simulink model "BEV_Laengsdynamikmodell_Reiter"  (R2022b)
settings: Solver=FixedStepAuto  StartTime=0.0  StopTime=1068  FixedStep=0.001  MaxStep=0.1  RelTol=1e-3  EnableMultiTasking=on
model workspace (MAT data in the model file):
  BTMSConfig.BTMS_included = 1
  BTMSConfig.T_fluid = 20
  BTMSConfig.Vdot_BTMS = 0.0045
  BTMSConfig.channel_def_mat = [1  2  3  0  0  0; 334  335  336  0  0  0; 10  11  12  13  14  15; 19  20  21  22  23  24; 28  29  30  31  32  33; 52  53  54  55  56  57; 61  62  63  64  65  66; 70  71  72  73  74  75; 94  95  96  97  98  99; 103  104  105  106  107  108; 112  113  114  115  116  117; 136  137  138  139  140  141; 145  146  147  148  149  150; 154  155  156  157  158  159; 178  179  180  181  182  183; 187  188  189  190  191  192; 196  197  198  199  200  201; 220  221  222  223  224  225; 229  230  231  232  233  234; 238  239  240  241  242  243; 262  263  264  265  266  267; 271  272  273  274  275  276; 280  281  282  283  284  285; 304  305  306  307  308  309; 313  314  315  316  317  318; 322  323  324  325  326  327]
  BTMSConfig.channel_num_adj_cells = [3 3 6 6 6 6 6 6 6 6 6 6 6 6 6 6 6 6 6 6 6 6 6 6 6 6]
  BTMSConfig.num_channels = 26
  BTMSConfig.channel_length = [1.03690125; 1.03690125; 1.03690125; 1.03690125; 1.03690125; 1.03690125; 1.03690125; 1.03690125; 1.03690125; 1.03690125; 1.03690125; 1.03690125; 1.03690125; 1.03690125; 1.03690125; 1.03690125; 1.03690125; 1.03690125; 1.03690125; 1.03690125; 1.03690125; 1.03690125; 1.03690125; 1.03690125; 1.03690125; 1.03690125]
  BTMSConfig.channel_mdot = [0.184314576259; 0.184314576259; 0.184314576259; 0.184314576259; 0.184314576259; 0.184314576259; 0.184314576259; 0.184314576259; 0.184314576259; 0.184314576259; 0.184314576259; 0.184314576259; 0.184314576259; 0.184314576259; 0.184314576259; 0.184314576259; 0.184314576259; 0.184314576259; 0.184314576259; 0.184314576259; 0.184314576259; 0.184314576259; 0.184314576259; 0.184314576259; 0.184314576259; 0.184314576259]
  BTMSConfig.fluid_para.kin_vis = 3.46803646108e-06
  BTMSConfig.fluid_para.lambda = 0.389148353131
  BTMSConfig.fluid_para.rho = 1064.92866283
  BTMSConfig.fluid_para.cp = 3312.04190374
  BTMSConfig.fluid_para.Pr = 31.4329250552
  BTMSConfig.lambda_wall = 236
  BTMSConfig.channel_alpha = [597.661290321; 597.661290321; 668.795841133; 668.795841133; 668.795841133; 668.795841133; 668.795841133; 668.795841133; 668.795841133; 668.795841133; 668.795841133; 668.795841133; 668.795841133; 668.795841133; 668.795841133; 668.795841133; 668.795841133; 668.795841133; 668.795841133; 668.795841133; 668.795841133; 668.795841133; 668.795841133; 668.795841133; 668.795841133; 668.795841133]
  BTMSConfig.channel_orientation = [120 120 120 120 120 120 120 120 120 120 120 120 120 120 120 120 120 120 120 120 120 120 120 120 120 120]
  BatPara.electrical.C_A = 73.6
  BatPara.electrical.OCV.U = [3.071 3.168 3.237 3.287 3.317 3.326 3.333 3.339 3.346 3.352 3.36 3.407 3.46 3.504 3.537 3.56 3.581 3.601 3.621 3.645 3.672 3.707 3.767 3.806 3.84 3.872 3.904 3.938 3.978 4.024 4.068 4.086 4.103 4.122 4.148 4.184]
  BatPara.electrical.OCV.SOC = [-1.355e-05 0.0099 0.0199 0.0299 0.0399 0.0499 0.0599 0.0699 0.0799 0.0899 0.0999 0.1399 0.1799 0.2199 0.2599 0.2999 0.3399 0.3799 0.4199 0.4599 0.4999 0.5399 0.5799 0.6199 0.6599 0.6999 0.7399 0.7799 0.8199 0.8599 0.8999 0.9199 0.9399 0.9599 0.9799 0.9999]
  BatPara.electrical.OCV.U_hyst = [0 0.0139 0.0165 0.0207 0.0196 0.0154 0.01449 0.0144 0.0144 0.0156 0.0186 0.0265 0.027 0.0307 0.0202 0.0156 0.0144 0.0144 0.0148 0.0162 0.0173 0.0171 0.0167 0.0148 0.0135 0.012 0.0112 0.0116 0.0122 0.0116 0.0095 0.008 0.0066 0.0062 0.004 -0.0013]
  BatPara.electrical.OCV.beta_hyst = 0.004
  BatPara.electrical.dyn.SOC = [0 0.1 0.2 0.3 0.4 0.5 0.6 0.7 0.8 0.9 1]
  BatPara.electrical.dyn.T = [8 25]
  BatPara.electrical.dyn.C_rate = [-1 1]
  BatPara.electrical.dyn.R_0 = reshape([0.00126739565217 0.00123344755435 0.00124099157609 0.00122590353261 0.00119195543478 0.00121081548913 0.0012145875 0.00118063940217 0.00116932336957 0.00118441141304 0.00121835951087 0.001041075 0.00101844293478 0.00101467092391 0.000995810869565 0.00100712690217 0.00100712690217 0.0010033548913 0.000995810869565 0.000999582880435 0.000999582880435 0.00101467092391 0.00126739565217 0.00123344755435 0.00123721956522 0.00124853559783 0.0012145875 0.00121835951087 0.00120327146739 0.00115423532609 0.00111651521739 0.00116177934783 0.00124853559783 0.00101844293478 0.0010033548913 0.000988266847826 0.000980722826087 0.000999582880435 0.00100712690217 0.000992038858696 0.000988266847826 0.000992038858696 0.000992038858696 0.00103353097826], [11 2 2])
  BatPara.electrical.dyn.RC1_enable = 1
  BatPara.electrical.dyn.R1 = reshape([0.00305155679348 0.00184074130435 0.000543169565217 0.0005205375 0.000535625543478 0.00052430951087 0.000595977717391 0.000675189945652 0.000656329891304 0.000671417934783 0.00310813695652 0.00144845217391 0.00026404076087 0.000324392934783 0.000441325271739 0.00043755326087 0.000467729347826 0.000543169565217 0.000577117663043 0.000622381793478 0.000716682065217 0.000392289130435 0.00228583858696 0.000531853532609 0.000558257608696 0.0005205375 0.000535625543478 0.000528081521739 0.000599749728261 0.000588433695652 0.000573345652174 0.00078457826087 0.00527327119565 0.00043000923913 0.000497905434783 0.000562029619565 0.000471501358696 0.00043000923913 0.000467729347826 0.000531853532609 0.000550713586957 0.000645013858696 0.000347025 0.00200293777174], [11 2 2])
  BatPara.electrical.dyn.C1 = reshape([479.653973057 217.512628773 46.5003962251 42.831265759 41.5216194799 46.4844895901 51.8132123046 53.3853180607 49.1037821483 56.1530725452 111.221842807 262.053857791 81.8714501837 106.455154528 100.415935451 100.681046034 103.313594121 101.874043657 100.628023918 97.120610907 102.99015921 115.718118291 136.505439089 54.5809667891 52.1048339457 51.0443916144 48.1758951084 49.1170376774 50.7023989626 41.7018946762 34.2814494633 86.0389885455 157.18936676 95.0819105252 125.646509617 106.444550104 88.175779843 87.666767524 98.570765795 90.2781067646 87.6057920899 95.423903177 88.220848642 173.719011599], [11 2 2])
  BatPara.electrical.dyn.RC2_enable = 1
  BatPara.electrical.dyn.R2 = reshape([0.0371128149457 0.00761568994565 0.00188223342391 0.00149371630435 0.00124099157609 0.00113914728261 0.00121835951087 0.00130888777174 0.0014371361413 0.00179170516304 0.00087133451087 0.00198784972826 0.00157292853261 0.000788350271739 0.000279128804348 0.000147108423913 0.000101844293478 0.000147108423913 0.000154652445652 0.000211232608696 0.000463957336957 0.00153143641304 0.00158801657609 0.00150503233696 0.00138432798913 0.0011768673913 0.00102598695652 0.000992038858696 0.0010901111413 0.00123344755435 0.0014371361413 0.0023801388587 0.00301760869565 0.00110142717391 0.000769490217391 0.000324392934783 0.000203688586957 0.000132020380435 8.29842391304e-05 0.000139564402174 0.000143336413043 0.0001735125 0.000943002717391 0.00147108423913], [11 2 2])
  BatPara.electrical.dyn.C2 = reshape([1973.40894748 900.304934803 341.260946618 299.415892227 291.865542828 295.05482314 288.522498379 273.085109142 245.8184857 221.216223615 7420.2702399 6327.38897774 467.140753548 432.665773359 969.97334486 2103.52257042 4757.71958793 4941.24503998 4682.62966645 2433.97495858 823.399005835 207.488797637 8423.5149629 263.172624451 257.859808371 259.540609466 269.651927095 270.137079461 266.825848282 219.021107989 196.134111375 206.189755781 753.934730927 364.492586989 467.445630718 1063.18622578 1300.61131042 2191.47565737 6693.27604639 4673.61590663 3457.28059938 2977.36946906 249.909141993 598.921922052], [11 2 2])
  BatPara.electrical.dyn.RC3_enable = 1
  BatPara.electrical.dyn.R3 = reshape([0.0586321369565 0.00301760869565 0.00136169592391 0.000377201086957 0.000245180706522 0.000237636684783 0.000354569021739 0.000418693206522 0.000414921195652 0.000543169565217 0.00268944375 0.0130285255435 0.00200293777174 0.000305532880435 0.000207460597826 0.000199916576087 0.000218776630435 0.000294216847826 0.000282900815217 0.000294216847826 0.000396061141304 0.000716682065217 0.00111274320652 0.000988266847826 0.000467729347826 0.000309304891304 0.000267812771739 0.00025649673913 0.000445097282609 0.000354569021739 0.000331936956522 0.000667645923913 0.00183319728261 0.000973178804348 0.000550713586957 0.000297988858696 0.000226320652174 0.000203688586957 0.000218776630435 0.000316848913043 0.000286672826087 0.000294216847826 0.000320620923913 0.000912826630435], [11 2 2])
  BatPara.electrical.dyn.C3 = reshape([1248.67084504 11155.8533247 2688.2213097 10360.5215763 20766.1119516 25866.8395649 25835.0262949 18441.0921403 17529.1117355 14689.7773936 21614.4658166 967.65362726 1686.10330668 11397.103955 28173.3016353 32765.0169296 33814.8548375 30797.8964052 26280.4120741 23409.2644622 20198.7753044 17645.7603919 110580.275196 12033.3693538 21842.4609178 32287.8178806 35262.3586197 33658.4395937 24832.9082919 30169.5843239 23600.1440818 8825.53130178 4782.59491391 11481.9393415 18952.7555652 32881.6655861 35774.0220445 36179.6412362 36784.093365 33279.3314603 34679.1153375 30267.6752395 14806.42605 10532.8434551], [11 2 2])
  BatPara.electrical.dyn.RC4_enable = 1
  BatPara.electrical.dyn.R4 = reshape([0.00299120461957 0.00170494891304 0.00207460597826 0.00211609809783 0.00188600543478 0.00175398505435 0.00305910081522 0.00309682092391 0.00262909157609 0.00293085244565 0.0235524358696 0.00224811847826 0.0018596013587 0.0014258201087 0.00130888777174 0.00113914728261 0.00103730298913 0.00235750679348 0.00175775706522 0.00150880434783 0.00162573668478 0.0036060423913 0.00636715434783 0.00329296548913 0.00247066711957 0.00219531032609 0.00185205733696 0.00163328070652 0.00284786820652 0.00268944375 0.00252724728261 0.00311190896739 0.00737805326087 0.00293839646739 0.00196144565217 0.00135792391304 0.00102975896739 0.0008675625 0.000886422554348 0.0019576736413 0.00150503233696 0.0014258201087 0.00169363288043 0.00431895244565], [11 2 2])
  BatPara.electrical.dyn.C4 = reshape([24482.9623226 39292.0394784 29930.9847994 32009.4517686 34382.1914848 35206.6853973 29949.5425402 24546.5888625 25394.9427275 24239.0605864 85967.4086881 14848.8437432 27059.8371875 39573.0566962 47080.9884014 52152.5538506 55116.4901664 39920.3515597 35811.1375261 35657.3733881 35720.999928 32825.9923637 19355.723651 33178.5894388 35596.397954 38769.7716303 40774.0076363 39631.3810244 31959.0807579 34273.4961458 29634.0609466 26036.5103379 17738.5490959 31012.6359772 48711.4184857 53045.9765147 53928.7947554 55034.3058857 59010.9646279 47931.9933722 52998.2566098 47555.5363446 33292.5869894 24984.0213241], [11 2 2])
  BatPara.electrical.U_max = 4.2
  BatPara.electrical.U_min = 2.5
  BatPara.electrical.U_nom = 3.6
  BatPara.electrical.I_max = 147.2
  BatPara.physical.m = 0.92076831
  BatPara.physical.A = 0.00418460141458
  BatPara.physical.rho = 2460.5
  BatPara.physical.c = 696.07
  BatPara.physical.dim_x = 0.007
  BatPara.physical.dim_y = 0.33
  BatPara.physical.dim_z = 0.162
  BatPara.physical.TabWidth = 0.04
  BatPara.physical.TabHeight = 0.03
  BatPara.thermal.EnCo = 0.0001
  BatPara.thermal.c = 700
  BatPara.thermal.A = 0.113808
  BatPara.variances.electrical.C_A = 0
  BatPara.variances.electrical.R_0 = 0
  BatPara.variances.electrical.R1 = 0
  BatPara.variances.electrical.C1 = 0
  BatPara.variances.electrical.R2 = 0
  BatPara.variances.electrical.C2 = 0
  BatPara.variances.electrical.R3 = 0
  BatPara.variances.electrical.C3 = 0
  BatPara.variances.electrical.R4 = 0
  BatPara.variances.electrical.C4 = 0
  BatPara.variances.physical.m = 0
  BatPara.variances.thermal.c = 0
  BatPara.variances.thermal.EnCo = 0
  SysPara.Balancing.R = 11
  SysPara.Balancing.U_Delta = 0.05
  SysPara.Balancing.U_Limit = 3.8
  SysPara.Balancing.I_Limit = 1.5
  SysPara.Balancing.t_Start = 0
  SysPara.p_mod = 3
  SysPara.s_mod = 14
  SysPara.thermal.transfer.A_x = 0.05346
  SysPara.thermal.transfer.A_y = 0.001134
  SysPara.thermal.transfer.A_z = 0.00231
  SysPara.thermal.transfer.alpha_x = 1000
  SysPara.thermal.transfer.alpha_y = 1000
  SysPara.thermal.transfer.alpha_z = 1000
  SysPara.thermal.transfer.alpha_mod_gap = 100
  SysPara.thermal.transfer.layer = [14 28 42 56 70 84 98]
  SysPara.thermal.transfer.dir = 'xxxxxxx'
  SysPara.thermal.transfer.alpha = [100 100 100 100 100 100 100]
  SysPara.thermal.transfer.K_transfer = [-54.594 1.134 0 53.46 0 0 0 0 0 0 0 0 ... (112896 elements, 336x336)]
  SysPara.thermal.T_cell_ambient = 25
  SysPara.thermal.alpha_cell_ambient = 0
  SysPara.pe_mod = 3
  SysPara.e_mod = 1
  SysPara.p_sys = 3
  SysPara.s_sys = 112
  SysPara.pe_sys = 3
  SysPara.e_sys = 1
  SysPara.I_charge_min = 10
  SysPara.SOC_charge_max = 1
  SysPara.p = 3
  SysPara.s = 112
  SysPara.I_charge = 40
  SysPara.U_charge_target = 4.18418
  SysPara.DeviationMap.C_A = [1  1  1  1  1  1  1  1  1  1  1  1  1  1  1  1  1  1  1  1  1  1  1  1  1  1  1  1  1  1  1  1  1  1  1  1  1  1  1  1  1  1  1  1  1  1  1  1  1  1  1  1  1  1  1  1  1  1  1  1  1  1  1  1  1  1  1  1  1  1  1  1  1  1  1  1  1  1  1  1  1  1  1  1  1  1  1  1  1  1  1  1  1  1  1  1  1  1  1  1  1  1  1  1  1  1  1  1  1  1  1  1; 1  1  1  1  1  1  1  1  1  1  1  1  1  1  1  1  1  1  1  1  1  1  1  1  1  1  1  1  1  1  1  1  1  1  1  1  1  1  1  1  1  1  1  1  1  1  1  1  1  1  1  1  1  1  1  1  1  1  1  1  1  1  1  1  1  1  1  1  1  1  1  1  1  1  1  1  1  1  1  1  1  1  1  1  1  1  1  1  1  1  1  1  1  1  1  1  1  1  1  1  1  1  1  1  1  1  1  1  1  1  1  1; 1  1  1  1  1  1  1  1  1  1  1  1  1  1  1  1  1  1  1  1  1  1  1  1  1  1  1  1  1  1  1  1  1  1  1  1  1  1  1  1  1  1  1  1  1  1  1  1  1  1  1  1  1  1  1  1  1  1  1  1  1  1  1  1  1  1  1  1  1  1  1  1  1  1  1  1  1  1  1  1  1  1  1  1  1  1  1  1  1  1  1  1  1  1  1  1  1  1  1  1  1  1  1  1  1  1  1  1  1  1  1  1]
  SysPara.DeviationMap.R_0 = [1  1  1  1  1  1  1  1  1  1  1  1  1  1  1  1  1  1  1  1  1  1  1  1  1  1  1  1  1  1  1  1  1  1  1  1  1  1  1  1  1  1  1  1  1  1  1  1  1  1  1  1  1  1  1  1  1  1  1  1  1  1  1  1  1  1  1  1  1  1  1  1  1  1  1  1  1  1  1  1  1  1  1  1  1  1  1  1  1  1  1  1  1  1  1  1  1  1  1  1  1  1  1  1  1  1  1  1  1  1  1  1; 1  1  1  1  1  1  1  1  1  1  1  1  1  1  1  1  1  1  1  1  1  1  1  1  1  1  1  1  1  1  1  1  1  1  1  1  1  1  1  1  1  1  1  1  1  1  1  1  1  1  1  1  1  1  1  1  1  1  1  1  1  1  1  1  1  1  1  1  1  1  1  1  1  1  1  1  1  1  1  1  1  1  1  1  1  1  1  1  1  1  1  1  1  1  1  1  1  1  1  1  1  1  1  1  1  1  1  1  1  1  1  1; 1  1  1  1  1  1  1  1  1  1  1  1  1  1  1  1  1  1  1  1  1  1  1  1  1  1  1  1  1  1  1  1  1  1  1  1  1  1  1  1  1  1  1  1  1  1  1  1  1  1  1  1  1  1  1  1  1  1  1  1  1  1  1  1  1  1  1  1  1  1  1  1  1  1  1  1  1  1  1  1  1  1  1  1  1  1  1  1  1  1  1  1  1  1  1  1  1  1  1  1  1  1  1  1  1  1  1  1  1  1  1  1]
  SysPara.DeviationMap.C1 = [1  1  1  1  1  1  1  1  1  1  1  1  1  1  1  1  1  1  1  1  1  1  1  1  1  1  1  1  1  1  1  1  1  1  1  1  1  1  1  1  1  1  1  1  1  1  1  1  1  1  1  1  1  1  1  1  1  1  1  1  1  1  1  1  1  1  1  1  1  1  1  1  1  1  1  1  1  1  1  1  1  1  1  1  1  1  1  1  1  1  1  1  1  1  1  1  1  1  1  1  1  1  1  1  1  1  1  1  1  1  1  1; 1  1  1  1  1  1  1  1  1  1  1  1  1  1  1  1  1  1  1  1  1  1  1  1  1  1  1  1  1  1  1  1  1  1  1  1  1  1  1  1  1  1  1  1  1  1  1  1  1  1  1  1  1  1  1  1  1  1  1  1  1  1  1  1  1  1  1  1  1  1  1  1  1  1  1  1  1  1  1  1  1  1  1  1  1  1  1  1  1  1  1  1  1  1  1  1  1  1  1  1  1  1  1  1  1  1  1  1  1  1  1  1; 1  1  1  1  1  1  1  1  1  1  1  1  1  1  1  1  1  1  1  1  1  1  1  1  1  1  1  1  1  1  1  1  1  1  1  1  1  1  1  1  1  1  1  1  1  1  1  1  1  1  1  1  1  1  1  1  1  1  1  1  1  1  1  1  1  1  1  1  1  1  1  1  1  1  1  1  1  1  1  1  1  1  1  1  1  1  1  1  1  1  1  1  1  1  1  1  1  1  1  1  1  1  1  1  1  1  1  1  1  1  1  1]
  SysPara.DeviationMap.C2 = [1  1  1  1  1  1  1  1  1  1  1  1  1  1  1  1  1  1  1  1  1  1  1  1  1  1  1  1  1  1  1  1  1  1  1  1  1  1  1  1  1  1  1  1  1  1  1  1  1  1  1  1  1  1  1  1  1  1  1  1  1  1  1  1  1  1  1  1  1  1  1  1  1  1  1  1  1  1  1  1  1  1  1  1  1  1  1  1  1  1  1  1  1  1  1  1  1  1  1  1  1  1  1  1  1  1  1  1  1  1  1  1; 1  1  1  1  1  1  1  1  1  1  1  1  1  1  1  1  1  1  1  1  1  1  1  1  1  1  1  1  1  1  1  1  1  1  1  1  1  1  1  1  1  1  1  1  1  1  1  1  1  1  1  1  1  1  1  1  1  1  1  1  1  1  1  1  1  1  1  1  1  1  1  1  1  1  1  1  1  1  1  1  1  1  1  1  1  1  1  1  1  1  1  1  1  1  1  1  1  1  1  1  1  1  1  1  1  1  1  1  1  1  1  1; 1  1  1  1  1  1  1  1  1  1  1  1  1  1  1  1  1  1  1  1  1  1  1  1  1  1  1  1  1  1  1  1  1  1  1  1  1  1  1  1  1  1  1  1  1  1  1  1  1  1  1  1  1  1  1  1  1  1  1  1  1  1  1  1  1  1  1  1  1  1  1  1  1  1  1  1  1  1  1  1  1  1  1  1  1  1  1  1  1  1  1  1  1  1  1  1  1  1  1  1  1  1  1  1  1  1  1  1  1  1  1  1]
  SysPara.DeviationMap.C3 = [1  1  1  1  1  1  1  1  1  1  1  1  1  1  1  1  1  1  1  1  1  1  1  1  1  1  1  1  1  1  1  1  1  1  1  1  1  1  1  1  1  1  1  1  1  1  1  1  1  1  1  1  1  1  1  1  1  1  1  1  1  1  1  1  1  1  1  1  1  1  1  1  1  1  1  1  1  1  1  1  1  1  1  1  1  1  1  1  1  1  1  1  1  1  1  1  1  1  1  1  1  1  1  1  1  1  1  1  1  1  1  1; 1  1  1  1  1  1  1  1  1  1  1  1  1  1  1  1  1  1  1  1  1  1  1  1  1  1  1  1  1  1  1  1  1  1  1  1  1  1  1  1  1  1  1  1  1  1  1  1  1  1  1  1  1  1  1  1  1  1  1  1  1  1  1  1  1  1  1  1  1  1  1  1  1  1  1  1  1  1  1  1  1  1  1  1  1  1  1  1  1  1  1  1  1  1  1  1  1  1  1  1  1  1  1  1  1  1  1  1  1  1  1  1; 1  1  1  1  1  1  1  1  1  1  1  1  1  1  1  1  1  1  1  1  1  1  1  1  1  1  1  1  1  1  1  1  1  1  1  1  1  1  1  1  1  1  1  1  1  1  1  1  1  1  1  1  1  1  1  1  1  1  1  1  1  1  1  1  1  1  1  1  1  1  1  1  1  1  1  1  1  1  1  1  1  1  1  1  1  1  1  1  1  1  1  1  1  1  1  1  1  1  1  1  1  1  1  1  1  1  1  1  1  1  1  1]
  SysPara.DeviationMap.C4 = [1  1  1  1  1  1  1  1  1  1  1  1  1  1  1  1  1  1  1  1  1  1  1  1  1  1  1  1  1  1  1  1  1  1  1  1  1  1  1  1  1  1  1  1  1  1  1  1  1  1  1  1  1  1  1  1  1  1  1  1  1  1  1  1  1  1  1  1  1  1  1  1  1  1  1  1  1  1  1  1  1  1  1  1  1  1  1  1  1  1  1  1  1  1  1  1  1  1  1  1  1  1  1  1  1  1  1  1  1  1  1  1; 1  1  1  1  1  1  1  1  1  1  1  1  1  1  1  1  1  1  1  1  1  1  1  1  1  1  1  1  1  1  1  1  1  1  1  1  1  1  1  1  1  1  1  1  1  1  1  1  1  1  1  1  1  1  1  1  1  1  1  1  1  1  1  1  1  1  1  1  1  1  1  1  1  1  1  1  1  1  1  1  1  1  1  1  1  1  1  1  1  1  1  1  1  1  1  1  1  1  1  1  1  1  1  1  1  1  1  1  1  1  1  1; 1  1  1  1  1  1  1  1  1  1  1  1  1  1  1  1  1  1  1  1  1  1  1  1  1  1  1  1  1  1  1  1  1  1  1  1  1  1  1  1  1  1  1  1  1  1  1  1  1  1  1  1  1  1  1  1  1  1  1  1  1  1  1  1  1  1  1  1  1  1  1  1  1  1  1  1  1  1  1  1  1  1  1  1  1  1  1  1  1  1  1  1  1  1  1  1  1  1  1  1  1  1  1  1  1  1  1  1  1  1  1  1]
  SysPara.DeviationMap.R1 = [1  1  1  1  1  1  1  1  1  1  1  1  1  1  1  1  1  1  1  1  1  1  1  1  1  1  1  1  1  1  1  1  1  1  1  1  1  1  1  1  1  1  1  1  1  1  1  1  1  1  1  1  1  1  1  1  1  1  1  1  1  1  1  1  1  1  1  1  1  1  1  1  1  1  1  1  1  1  1  1  1  1  1  1  1  1  1  1  1  1  1  1  1  1  1  1  1  1  1  1  1  1  1  1  1  1  1  1  1  1  1  1; 1  1  1  1  1  1  1  1  1  1  1  1  1  1  1  1  1  1  1  1  1  1  1  1  1  1  1  1  1  1  1  1  1  1  1  1  1  1  1  1  1  1  1  1  1  1  1  1  1  1  1  1  1  1  1  1  1  1  1  1  1  1  1  1  1  1  1  1  1  1  1  1  1  1  1  1  1  1  1  1  1  1  1  1  1  1  1  1  1  1  1  1  1  1  1  1  1  1  1  1  1  1  1  1  1  1  1  1  1  1  1  1; 1  1  1  1  1  1  1  1  1  1  1  1  1  1  1  1  1  1  1  1  1  1  1  1  1  1  1  1  1  1  1  1  1  1  1  1  1  1  1  1  1  1  1  1  1  1  1  1  1  1  1  1  1  1  1  1  1  1  1  1  1  1  1  1  1  1  1  1  1  1  1  1  1  1  1  1  1  1  1  1  1  1  1  1  1  1  1  1  1  1  1  1  1  1  1  1  1  1  1  1  1  1  1  1  1  1  1  1  1  1  1  1]
  SysPara.DeviationMap.R2 = [1  1  1  1  1  1  1  1  1  1  1  1  1  1  1  1  1  1  1  1  1  1  1  1  1  1  1  1  1  1  1  1  1  1  1  1  1  1  1  1  1  1  1  1  1  1  1  1  1  1  1  1  1  1  1  1  1  1  1  1  1  1  1  1  1  1  1  1  1  1  1  1  1  1  1  1  1  1  1  1  1  1  1  1  1  1  1  1  1  1  1  1  1  1  1  1  1  1  1  1  1  1  1  1  1  1  1  1  1  1  1  1; 1  1  1  1  1  1  1  1  1  1  1  1  1  1  1  1  1  1  1  1  1  1  1  1  1  1  1  1  1  1  1  1  1  1  1  1  1  1  1  1  1  1  1  1  1  1  1  1  1  1  1  1  1  1  1  1  1  1  1  1  1  1  1  1  1  1  1  1  1  1  1  1  1  1  1  1  1  1  1  1  1  1  1  1  1  1  1  1  1  1  1  1  1  1  1  1  1  1  1  1  1  1  1  1  1  1  1  1  1  1  1  1; 1  1  1  1  1  1  1  1  1  1  1  1  1  1  1  1  1  1  1  1  1  1  1  1  1  1  1  1  1  1  1  1  1  1  1  1  1  1  1  1  1  1  1  1  1  1  1  1  1  1  1  1  1  1  1  1  1  1  1  1  1  1  1  1  1  1  1  1  1  1  1  1  1  1  1  1  1  1  1  1  1  1  1  1  1  1  1  1  1  1  1  1  1  1  1  1  1  1  1  1  1  1  1  1  1  1  1  1  1  1  1  1]
  SysPara.DeviationMap.R3 = [1  1  1  1  1  1  1  1  1  1  1  1  1  1  1  1  1  1  1  1  1  1  1  1  1  1  1  1  1  1  1  1  1  1  1  1  1  1  1  1  1  1  1  1  1  1  1  1  1  1  1  1  1  1  1  1  1  1  1  1  1  1  1  1  1  1  1  1  1  1  1  1  1  1  1  1  1  1  1  1  1  1  1  1  1  1  1  1  1  1  1  1  1  1  1  1  1  1  1  1  1  1  1  1  1  1  1  1  1  1  1  1; 1  1  1  1  1  1  1  1  1  1  1  1  1  1  1  1  1  1  1  1  1  1  1  1  1  1  1  1  1  1  1  1  1  1  1  1  1  1  1  1  1  1  1  1  1  1  1  1  1  1  1  1  1  1  1  1  1  1  1  1  1  1  1  1  1  1  1  1  1  1  1  1  1  1  1  1  1  1  1  1  1  1  1  1  1  1  1  1  1  1  1  1  1  1  1  1  1  1  1  1  1  1  1  1  1  1  1  1  1  1  1  1; 1  1  1  1  1  1  1  1  1  1  1  1  1  1  1  1  1  1  1  1  1  1  1  1  1  1  1  1  1  1  1  1  1  1  1  1  1  1  1  1  1  1  1  1  1  1  1  1  1  1  1  1  1  1  1  1  1  1  1  1  1  1  1  1  1  1  1  1  1  1  1  1  1  1  1  1  1  1  1  1  1  1  1  1  1  1  1  1  1  1  1  1  1  1  1  1  1  1  1  1  1  1  1  1  1  1  1  1  1  1  1  1]
  SysPara.DeviationMap.R4 = [1  1  1  1  1  1  1  1  1  1  1  1  1  1  1  1  1  1  1  1  1  1  1  1  1  1  1  1  1  1  1  1  1  1  1  1  1  1  1  1  1  1  1  1  1  1  1  1  1  1  1  1  1  1  1  1  1  1  1  1  1  1  1  1  1  1  1  1  1  1  1  1  1  1  1  1  1  1  1  1  1  1  1  1  1  1  1  1  1  1  1  1  1  1  1  1  1  1  1  1  1  1  1  1  1  1  1  1  1  1  1  1; 1  1  1  1  1  1  1  1  1  1  1  1  1  1  1  1  1  1  1  1  1  1  1  1  1  1  1  1  1  1  1  1  1  1  1  1  1  1  1  1  1  1  1  1  1  1  1  1  1  1  1  1  1  1  1  1  1  1  1  1  1  1  1  1  1  1  1  1  1  1  1  1  1  1  1  1  1  1  1  1  1  1  1  1  1  1  1  1  1  1  1  1  1  1  1  1  1  1  1  1  1  1  1  1  1  1  1  1  1  1  1  1; 1  1  1  1  1  1  1  1  1  1  1  1  1  1  1  1  1  1  1  1  1  1  1  1  1  1  1  1  1  1  1  1  1  1  1  1  1  1  1  1  1  1  1  1  1  1  1  1  1  1  1  1  1  1  1  1  1  1  1  1  1  1  1  1  1  1  1  1  1  1  1  1  1  1  1  1  1  1  1  1  1  1  1  1  1  1  1  1  1  1  1  1  1  1  1  1  1  1  1  1  1  1  1  1  1  1  1  1  1  1  1  1]
  SysPara.DeviationMap.m = [1  1  1  1  1  1  1  1  1  1  1  1  1  1  1  1  1  1  1  1  1  1  1  1  1  1  1  1  1  1  1  1  1  1  1  1  1  1  1  1  1  1  1  1  1  1  1  1  1  1  1  1  1  1  1  1  1  1  1  1  1  1  1  1  1  1  1  1  1  1  1  1  1  1  1  1  1  1  1  1  1  1  1  1  1  1  1  1  1  1  1  1  1  1  1  1  1  1  1  1  1  1  1  1  1  1  1  1  1  1  1  1; 1  1  1  1  1  1  1  1  1  1  1  1  1  1  1  1  1  1  1  1  1  1  1  1  1  1  1  1  1  1  1  1  1  1  1  1  1  1  1  1  1  1  1  1  1  1  1  1  1  1  1  1  1  1  1  1  1  1  1  1  1  1  1  1  1  1  1  1  1  1  1  1  1  1  1  1  1  1  1  1  1  1  1  1  1  1  1  1  1  1  1  1  1  1  1  1  1  1  1  1  1  1  1  1  1  1  1  1  1  1  1  1; 1  1  1  1  1  1  1  1  1  1  1  1  1  1  1  1  1  1  1  1  1  1  1  1  1  1  1  1  1  1  1  1  1  1  1  1  1  1  1  1  1  1  1  1  1  1  1  1  1  1  1  1  1  1  1  1  1  1  1  1  1  1  1  1  1  1  1  1  1  1  1  1  1  1  1  1  1  1  1  1  1  1  1  1  1  1  1  1  1  1  1  1  1  1  1  1  1  1  1  1  1  1  1  1  1  1  1  1  1  1  1  1]
  SysPara.DeviationMap.c = [1  1  1  1  1  1  1  1  1  1  1  1  1  1  1  1  1  1  1  1  1  1  1  1  1  1  1  1  1  1  1  1  1  1  1  1  1  1  1  1  1  1  1  1  1  1  1  1  1  1  1  1  1  1  1  1  1  1  1  1  1  1  1  1  1  1  1  1  1  1  1  1  1  1  1  1  1  1  1  1  1  1  1  1  1  1  1  1  1  1  1  1  1  1  1  1  1  1  1  1  1  1  1  1  1  1  1  1  1  1  1  1; 1  1  1  1  1  1  1  1  1  1  1  1  1  1  1  1  1  1  1  1  1  1  1  1  1  1  1  1  1  1  1  1  1  1  1  1  1  1  1  1  1  1  1  1  1  1  1  1  1  1  1  1  1  1  1  1  1  1  1  1  1  1  1  1  1  1  1  1  1  1  1  1  1  1  1  1  1  1  1  1  1  1  1  1  1  1  1  1  1  1  1  1  1  1  1  1  1  1  1  1  1  1  1  1  1  1  1  1  1  1  1  1; 1  1  1  1  1  1  1  1  1  1  1  1  1  1  1  1  1  1  1  1  1  1  1  1  1  1  1  1  1  1  1  1  1  1  1  1  1  1  1  1  1  1  1  1  1  1  1  1  1  1  1  1  1  1  1  1  1  1  1  1  1  1  1  1  1  1  1  1  1  1  1  1  1  1  1  1  1  1  1  1  1  1  1  1  1  1  1  1  1  1  1  1  1  1  1  1  1  1  1  1  1  1  1  1  1  1  1  1  1  1  1  1]
  SysPara.DeviationMap.EnCo = [1  1  1  1  1  1  1  1  1  1  1  1  1  1  1  1  1  1  1  1  1  1  1  1  1  1  1  1  1  1  1  1  1  1  1  1  1  1  1  1  1  1  1  1  1  1  1  1  1  1  1  1  1  1  1  1  1  1  1  1  1  1  1  1  1  1  1  1  1  1  1  1  1  1  1  1  1  1  1  1  1  1  1  1  1  1  1  1  1  1  1  1  1  1  1  1  1  1  1  1  1  1  1  1  1  1  1  1  1  1  1  1; 1  1  1  1  1  1  1  1  1  1  1  1  1  1  1  1  1  1  1  1  1  1  1  1  1  1  1  1  1  1  1  1  1  1  1  1  1  1  1  1  1  1  1  1  1  1  1  1  1  1  1  1  1  1  1  1  1  1  1  1  1  1  1  1  1  1  1  1  1  1  1  1  1  1  1  1  1  1  1  1  1  1  1  1  1  1  1  1  1  1  1  1  1  1  1  1  1  1  1  1  1  1  1  1  1  1  1  1  1  1  1  1; 1  1  1  1  1  1  1  1  1  1  1  1  1  1  1  1  1  1  1  1  1  1  1  1  1  1  1  1  1  1  1  1  1  1  1  1  1  1  1  1  1  1  1  1  1  1  1  1  1  1  1  1  1  1  1  1  1  1  1  1  1  1  1  1  1  1  1  1  1  1  1  1  1  1  1  1  1  1  1  1  1  1  1  1  1  1  1  1  1  1  1  1  1  1  1  1  1  1  1  1  1  1  1  1  1  1  1  1  1  1  1  1]
  SysPara.BatStateInit.electrical.SOC = [0.05 0.05 0.05 0.05 0.05 0.05 0.05 0.05 0.05 0.05 0.05 0.05 ... (336 elements, 3x112)]
  SysPara.BatStateInit.electrical.U_hyst = [0  0  0  0  0  0  0  0  0  0  0  0  0  0  0  0  0  0  0  0  0  0  0  0  0  0  0  0  0  0  0  0  0  0  0  0  0  0  0  0  0  0  0  0  0  0  0  0  0  0  0  0  0  0  0  0  0  0  0  0  0  0  0  0  0  0  0  0  0  0  0  0  0  0  0  0  0  0  0  0  0  0  0  0  0  0  0  0  0  0  0  0  0  0  0  0  0  0  0  0  0  0  0  0  0  0  0  0  0  0  0  0; 0  0  0  0  0  0  0  0  0  0  0  0  0  0  0  0  0  0  0  0  0  0  0  0  0  0  0  0  0  0  0  0  0  0  0  0  0  0  0  0  0  0  0  0  0  0  0  0  0  0  0  0  0  0  0  0  0  0  0  0  0  0  0  0  0  0  0  0  0  0  0  0  0  0  0  0  0  0  0  0  0  0  0  0  0  0  0  0  0  0  0  0  0  0  0  0  0  0  0  0  0  0  0  0  0  0  0  0  0  0  0  0; 0  0  0  0  0  0  0  0  0  0  0  0  0  0  0  0  0  0  0  0  0  0  0  0  0  0  0  0  0  0  0  0  0  0  0  0  0  0  0  0  0  0  0  0  0  0  0  0  0  0  0  0  0  0  0  0  0  0  0  0  0  0  0  0  0  0  0  0  0  0  0  0  0  0  0  0  0  0  0  0  0  0  0  0  0  0  0  0  0  0  0  0  0  0  0  0  0  0  0  0  0  0  0  0  0  0  0  0  0  0  0  0]
  SysPara.BatStateInit.electrical.U_RC1 = [0  0  0  0  0  0  0  0  0  0  0  0  0  0  0  0  0  0  0  0  0  0  0  0  0  0  0  0  0  0  0  0  0  0  0  0  0  0  0  0  0  0  0  0  0  0  0  0  0  0  0  0  0  0  0  0  0  0  0  0  0  0  0  0  0  0  0  0  0  0  0  0  0  0  0  0  0  0  0  0  0  0  0  0  0  0  0  0  0  0  0  0  0  0  0  0  0  0  0  0  0  0  0  0  0  0  0  0  0  0  0  0; 0  0  0  0  0  0  0  0  0  0  0  0  0  0  0  0  0  0  0  0  0  0  0  0  0  0  0  0  0  0  0  0  0  0  0  0  0  0  0  0  0  0  0  0  0  0  0  0  0  0  0  0  0  0  0  0  0  0  0  0  0  0  0  0  0  0  0  0  0  0  0  0  0  0  0  0  0  0  0  0  0  0  0  0  0  0  0  0  0  0  0  0  0  0  0  0  0  0  0  0  0  0  0  0  0  0  0  0  0  0  0  0; 0  0  0  0  0  0  0  0  0  0  0  0  0  0  0  0  0  0  0  0  0  0  0  0  0  0  0  0  0  0  0  0  0  0  0  0  0  0  0  0  0  0  0  0  0  0  0  0  0  0  0  0  0  0  0  0  0  0  0  0  0  0  0  0  0  0  0  0  0  0  0  0  0  0  0  0  0  0  0  0  0  0  0  0  0  0  0  0  0  0  0  0  0  0  0  0  0  0  0  0  0  0  0  0  0  0  0  0  0  0  0  0]
  SysPara.BatStateInit.electrical.U_RC2 = [0  0  0  0  0  0  0  0  0  0  0  0  0  0  0  0  0  0  0  0  0  0  0  0  0  0  0  0  0  0  0  0  0  0  0  0  0  0  0  0  0  0  0  0  0  0  0  0  0  0  0  0  0  0  0  0  0  0  0  0  0  0  0  0  0  0  0  0  0  0  0  0  0  0  0  0  0  0  0  0  0  0  0  0  0  0  0  0  0  0  0  0  0  0  0  0  0  0  0  0  0  0  0  0  0  0  0  0  0  0  0  0; 0  0  0  0  0  0  0  0  0  0  0  0  0  0  0  0  0  0  0  0  0  0  0  0  0  0  0  0  0  0  0  0  0  0  0  0  0  0  0  0  0  0  0  0  0  0  0  0  0  0  0  0  0  0  0  0  0  0  0  0  0  0  0  0  0  0  0  0  0  0  0  0  0  0  0  0  0  0  0  0  0  0  0  0  0  0  0  0  0  0  0  0  0  0  0  0  0  0  0  0  0  0  0  0  0  0  0  0  0  0  0  0; 0  0  0  0  0  0  0  0  0  0  0  0  0  0  0  0  0  0  0  0  0  0  0  0  0  0  0  0  0  0  0  0  0  0  0  0  0  0  0  0  0  0  0  0  0  0  0  0  0  0  0  0  0  0  0  0  0  0  0  0  0  0  0  0  0  0  0  0  0  0  0  0  0  0  0  0  0  0  0  0  0  0  0  0  0  0  0  0  0  0  0  0  0  0  0  0  0  0  0  0  0  0  0  0  0  0  0  0  0  0  0  0]
  SysPara.BatStateInit.electrical.U_RC3 = [0  0  0  0  0  0  0  0  0  0  0  0  0  0  0  0  0  0  0  0  0  0  0  0  0  0  0  0  0  0  0  0  0  0  0  0  0  0  0  0  0  0  0  0  0  0  0  0  0  0  0  0  0  0  0  0  0  0  0  0  0  0  0  0  0  0  0  0  0  0  0  0  0  0  0  0  0  0  0  0  0  0  0  0  0  0  0  0  0  0  0  0  0  0  0  0  0  0  0  0  0  0  0  0  0  0  0  0  0  0  0  0; 0  0  0  0  0  0  0  0  0  0  0  0  0  0  0  0  0  0  0  0  0  0  0  0  0  0  0  0  0  0  0  0  0  0  0  0  0  0  0  0  0  0  0  0  0  0  0  0  0  0  0  0  0  0  0  0  0  0  0  0  0  0  0  0  0  0  0  0  0  0  0  0  0  0  0  0  0  0  0  0  0  0  0  0  0  0  0  0  0  0  0  0  0  0  0  0  0  0  0  0  0  0  0  0  0  0  0  0  0  0  0  0; 0  0  0  0  0  0  0  0  0  0  0  0  0  0  0  0  0  0  0  0  0  0  0  0  0  0  0  0  0  0  0  0  0  0  0  0  0  0  0  0  0  0  0  0  0  0  0  0  0  0  0  0  0  0  0  0  0  0  0  0  0  0  0  0  0  0  0  0  0  0  0  0  0  0  0  0  0  0  0  0  0  0  0  0  0  0  0  0  0  0  0  0  0  0  0  0  0  0  0  0  0  0  0  0  0  0  0  0  0  0  0  0]
  SysPara.BatStateInit.electrical.U_RC4 = [0  0  0  0  0  0  0  0  0  0  0  0  0  0  0  0  0  0  0  0  0  0  0  0  0  0  0  0  0  0  0  0  0  0  0  0  0  0  0  0  0  0  0  0  0  0  0  0  0  0  0  0  0  0  0  0  0  0  0  0  0  0  0  0  0  0  0  0  0  0  0  0  0  0  0  0  0  0  0  0  0  0  0  0  0  0  0  0  0  0  0  0  0  0  0  0  0  0  0  0  0  0  0  0  0  0  0  0  0  0  0  0; 0  0  0  0  0  0  0  0  0  0  0  0  0  0  0  0  0  0  0  0  0  0  0  0  0  0  0  0  0  0  0  0  0  0  0  0  0  0  0  0  0  0  0  0  0  0  0  0  0  0  0  0  0  0  0  0  0  0  0  0  0  0  0  0  0  0  0  0  0  0  0  0  0  0  0  0  0  0  0  0  0  0  0  0  0  0  0  0  0  0  0  0  0  0  0  0  0  0  0  0  0  0  0  0  0  0  0  0  0  0  0  0; 0  0  0  0  0  0  0  0  0  0  0  0  0  0  0  0  0  0  0  0  0  0  0  0  0  0  0  0  0  0  0  0  0  0  0  0  0  0  0  0  0  0  0  0  0  0  0  0  0  0  0  0  0  0  0  0  0  0  0  0  0  0  0  0  0  0  0  0  0  0  0  0  0  0  0  0  0  0  0  0  0  0  0  0  0  0  0  0  0  0  0  0  0  0  0  0  0  0  0  0  0  0  0  0  0  0  0  0  0  0  0  0]
  SysPara.BatStateInit.electrical.I_cell = [0  0  0  0  0  0  0  0  0  0  0  0  0  0  0  0  0  0  0  0  0  0  0  0  0  0  0  0  0  0  0  0  0  0  0  0  0  0  0  0  0  0  0  0  0  0  0  0  0  0  0  0  0  0  0  0  0  0  0  0  0  0  0  0  0  0  0  0  0  0  0  0  0  0  0  0  0  0  0  0  0  0  0  0  0  0  0  0  0  0  0  0  0  0  0  0  0  0  0  0  0  0  0  0  0  0  0  0  0  0  0  0; 0  0  0  0  0  0  0  0  0  0  0  0  0  0  0  0  0  0  0  0  0  0  0  0  0  0  0  0  0  0  0  0  0  0  0  0  0  0  0  0  0  0  0  0  0  0  0  0  0  0  0  0  0  0  0  0  0  0  0  0  0  0  0  0  0  0  0  0  0  0  0  0  0  0  0  0  0  0  0  0  0  0  0  0  0  0  0  0  0  0  0  0  0  0  0  0  0  0  0  0  0  0  0  0  0  0  0  0  0  0  0  0; 0  0  0  0  0  0  0  0  0  0  0  0  0  0  0  0  0  0  0  0  0  0  0  0  0  0  0  0  0  0  0  0  0  0  0  0  0  0  0  0  0  0  0  0  0  0  0  0  0  0  0  0  0  0  0  0  0  0  0  0  0  0  0  0  0  0  0  0  0  0  0  0  0  0  0  0  0  0  0  0  0  0  0  0  0  0  0  0  0  0  0  0  0  0  0  0  0  0  0  0  0  0  0  0  0  0  0  0  0  0  0  0]
  SysPara.BatStateInit.thermal.T_cell = [25  25  25  25  25  25  25  25  25  25  25  25  25  25  25  25  25  25  25  25  25  25  25  25  25  25  25  25  25  25  25  25  25  25  25  25  25  25  25  25  25  25  25  25  25  25  25  25  25  25  25  25  25  25  25  25  25  25  25  25  25  25  25  25  25  25  25  25  25  25  25  25  25  25  25  25  25  25  25  25  25  25  25  25  25  25  25  25  25  25  25  25  25  25  25  25  25  25  25  25  25  25  25  25  25  25  25  25  25  25  25  25; 25  25  25  25  25  25  25  25  25  25  25  25  25  25  25  25  25  25  25  25  25  25  25  25  25  25  25  25  25  25  25  25  25  25  25  25  25  25  25  25  25  25  25  25  25  25  25  25  25  25  25  25  25  25  25  25  25  25  25  25  25  25  25  25  25  25  25  25  25  25  25  25  25  25  25  25  25  25  25  25  25  25  25  25  25  25  25  25  25  25  25  25  25  25  25  25  25  25  25  25  25  25  25  25  25  25  25  25  25  25  25  25; 25  25  25  25  25  25  25  25  25  25  25  25  25  25  25  25  25  25  25  25  25  25  25  25  25  25  25  25  25  25  25  25  25  25  25  25  25  25  25  25  25  25  25  25  25  25  25  25  25  25  25  25  25  25  25  25  25  25  25  25  25  25  25  25  25  25  25  25  25  25  25  25  25  25  25  25  25  25  25  25  25  25  25  25  25  25  25  25  25  25  25  25  25  25  25  25  25  25  25  25  25  25  25  25  25  25  25  25  25  25  25  25]
undefined symbols (not defined in the file): gear_ratio, xC, yC, zC
settings Model: Creator=maximilian.tschochne  LastModifiedBy=ga84jar
settings SolverCC: AlgebraicLoopSolver=TrustRegion  AutoInsertRateTranBlk=on
settings DataIOCC: LimitDataPoints=on  SaveFormat=Array  SignalLoggingSaveFormat=ModelDataLogs  ReturnWorkspaceOutputs=off
settings OptimizationCC: BlockReduction=off  OptimizeBlockIOStorage=off  BufferReuse=off  GlobalBufferReuse=off  ExpressionFolding=off  ExpressionDepthLimit=2147483647  LocalBlockOutputs=off  LifeSpan=inf
settings DebuggingCC: UnderspecifiedInitializationDetection=Classic  MergeDetectMultiDrivingBlocksExec=none  SolverPrmCheckMsg=warning  FcnCallInpInsideContextMsg=warning  UnconnectedInputMsg=warning  UnconnectedOutputMsg=warning  UnconnectedLineMsg=warning  StateNameClashWarn=warning  SFUnexpectedBacktrackingDiag=warning  SFNoUnconditionalDefaultTransitionDiag=warning  SFExecutionAtInitializationDiag=none  SFMachineParentedDataDiag=warning  ArithmeticOperatorsInVariantConditions=warning
settings HardwareCC: ProdBitPerPointer=32  ProdBitPerSizeT=32  ProdBitPerPtrDiffT=32  ProdLargestAtomicFloat=None  ProdEndianess=BigEndian  ProdWordSize=32  ProdHWDeviceType=Generic->Custom  TargetIntDivRoundTo=Zero  TargetEndianess=BigEndian  TargetHWDeviceType=Generic->Custom
settings ModelReferenceCC: EnableRefExpFcnMdlSchedulingChecks=on  PropagateSignalLabelsOutOfModel=off
settings SFSimCC: SimUseLocalCustomCode=off  CustomCodeUndefinedFunction=UseInterfaceOnly
settings RTWCC: Description=dSPACE DS1401 Hardware Platform  SystemTargetFile=rti1401.tlc  MakeCommand=make_rti  TemplateMakefile=rti1401.tmf  RTWUseLocalCustomCode=off
settings CodeAppCC: StateflowObjectComments=on
settings STFCustomTargetCC: ParMdlRefBuildCompliant=on  MatFileLogging=on  CPPClassGenCompliant=on  GRTInterface=on  SystemTargetFile=rti1401.tlc
settings GRTTargetCC: TargetLangStandard=C89/C90 (ANSI)  CompOptLevelCompliant=off  ConcurrentExecutionCompliant=off  CombineOutputUpdateFcns=off  GRTInterface=on  UseToolchainInfoCompliant=off  ExtModeMexFile=noextcomm
settings ConfigComp: CovMetricSettings=dw  CovSaveCumulativeToWorkspaceVar=on  CovSaveSingleToWorkspaceVar=on  CovExternalEMLEnable=off  CovSFcnEnable=off  DVTestSuiteOptimization=Auto  DVDetectOutOfBounds=on  DVModelReferenceHarness=on  DVHarnessSource=Signal Editor

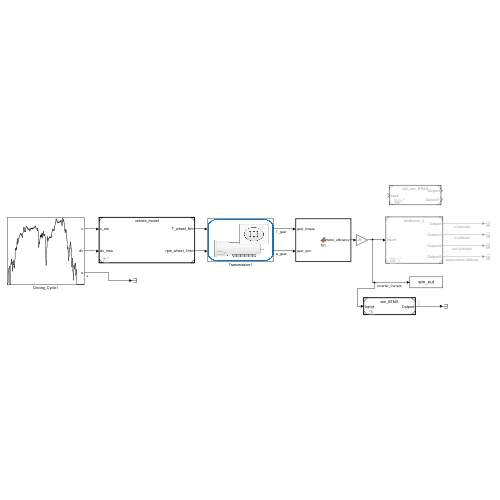
[thumbnail: Simulink's stored preview of the top-level diagram]
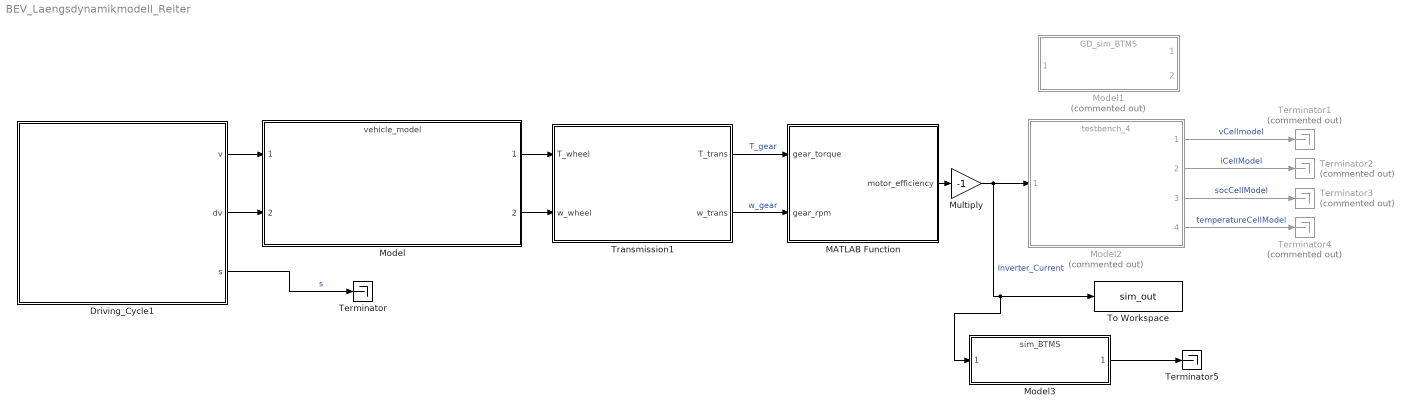
== system BEV_Laengsdynamikmodell_Reiter ==
  Driving_Cycle1 : Subsystem  mask{dcname=EUROPE_ARTEMIS_MOTORWAY, ShowDCPlot=off}
      mask prompts: dcname "Choose Driving Cycle"; ShowDCPlot "Show DC Plot"
      mask init:
      | init_driving_cycle
      mask TypeOptions dcname: EUROPE_ARTEMIS_MOTORWAY | EUROPE_ARTEMIS_ROAD | EUROPE_ARTEMIS_URBAN | EUROPE_City | EUROPE_EUDC | EUROPE_NEDC | EUROPE_UDC | JAPAN_10_15_MODE | JAPAN_10_MODE | JAPAN_10_MODE_3 | JAPAN_11_MODE | JAPAN_11_MODE_4 | JAPAN_15_MODE | USA_CITY_I | USA_CITY_II | USA_FTP_72 | USA_FTP_75 | USA_FTP_HIGHWAY | USA_NECC | WLTP_class_3
      mask Display:
      | port_label('output',1,'v');
      | port_label('output',2,'dv');
      | port_label('output',3,'s');
      | plot(T_zplot, V_zplot);
  MATLAB Function : MATLAB Function  TreatAsAtomicUnit=on
  Model : ModelReference  ModelNameDialog=vehicle_model.slx  SimulationMode=Normal  ModelReferenceVersion=1.13
  Model1 : ModelReference  Commented=on  ModelNameDialog=GD_sim_BTMS.slx  SimulationMode=Normal  ModelReferenceVersion=5.2
  Model2 : ModelReference  Commented=on  ModelNameDialog=testbench_4.slx  SimulationMode=Normal  ModelReferenceVersion=1.17
  Model3 : ModelReference  ModelNameDialog=sim_BTMS.slx  SimulationMode=Normal  ModelReferenceVersion=5.1
  Multiply : Gain  Gain=-1
  Terminator : Terminator
  Terminator{1..4} (4 alike) : Terminator  Commented=on
  Terminator5 : Terminator
  To Workspace : ToWorkspace  VariableName=sim_out  SampleTime=-1
  Transmission1 : Subsystem  mask{i=gear_ratio, eta=0.95}
      mask prompts: i "Transmission Ratio"; eta "Tranmisstion Efficiency"
      mask Display: image('Transmission.png')
  wires:
  Driving_Cycle1/1(v) -> Model/1
  Driving_Cycle1/2(dv) -> Model/2
  Model/1 -> Transmission1/1(T_wheel)
  Transmission1/1(T_trans) -> MATLAB Function/1(gear_torque)  "T_gear"
  Transmission1/2(w_trans) -> MATLAB Function/2(gear_rpm)  "w_gear"
  Model/2 -> Transmission1/2(w_wheel)
  Multiply/1 -> Model2/1, Model3/1, To Workspace/1  "Inverter_Current"
  Driving_Cycle1/3(s) -> Terminator/1  "s"
  Model2/1 -> Terminator1/1  "vCellmodel"
  Model2/2 -> Terminator2/1  "iCellModel"
  Model2/3 -> Terminator3/1  "socCellModel"
  Model2/4 -> Terminator4/1  "temperatureCellModel"
  MATLAB Function/1(motor_efficiency) -> Multiply/1
  Model3/1 -> Terminator5/1

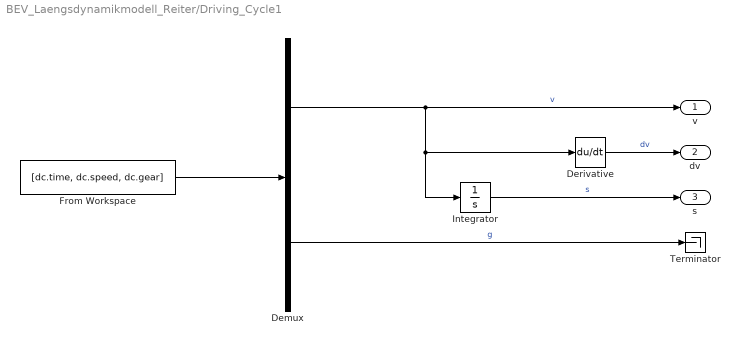
== system BEV_Laengsdynamikmodell_Reiter/Driving_Cycle1 ==
  Demux : Demux  Outputs=2
  Derivative : Derivative
  From Workspace : FromWorkspace  VariableName=[dc.time, dc.speed, dc.gear]
  Integrator : Integrator
  Terminator : Terminator
  v : Outport  VectorParamsAs1DForOutWhenUnconnected=off
  dv : Outport  Port=2  VectorParamsAs1DForOutWhenUnconnected=off
  s : Outport  Port=3  VectorParamsAs1DForOutWhenUnconnected=off
  wires:
  Integrator/1 -> s/1  "s"
  Demux/2 -> Terminator/1  "g"
  Derivative/1 -> dv/1  "dv"
  From Workspace/1 -> Demux/1
  Demux/1 -> v/1, Integrator/1, Derivative/1  "v"

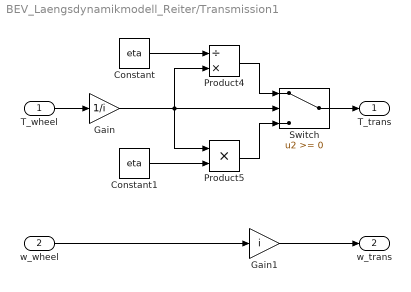
== system BEV_Laengsdynamikmodell_Reiter/Transmission1 ==
  T_wheel : Inport
  w_wheel : Inport  Port=2
  Constant : Constant  Value=eta
  Constant1 : Constant  Value=eta
  Gain : Gain  Gain=1/i
  Gain1 : Gain  Gain=i
  Product4 : Product  Inputs=/*  RndMeth=Zero
  Product5 : Product  RndMeth=Zero
  Switch : Switch  SaturateOnIntegerOverflow=off  InputSameDT=off
  T_trans : Outport  VectorParamsAs1DForOutWhenUnconnected=off
  w_trans : Outport  Port=2  VectorParamsAs1DForOutWhenUnconnected=off
  wires:
  T_wheel/1 -> Gain/1
  w_wheel/1 -> Gain1/1
  Gain1/1 -> w_trans/1
  Switch/1 -> T_trans/1
  Product4/1 -> Switch/1
  Product5/1 -> Switch/3
  Constant/1 -> Product4/1
  Constant1/1 -> Product5/2
  Gain/1 -> Switch/2, Product4/2, Product5/1

== matlab function BEV_Laengsdynamikmodell_Reiter/MATLAB Function ==
  data: gear_torque input; motor_efficiency output; gear_rpm input; xC parameter; yC parameter; zC parameter
function motor_efficiency = fcn(gear_torque, gear_rpm, xC, yC, zC)
    % this function calculates the efficency/current of the motor and electronics
    % from an efficiency map including motor torque and speed.

    diff_mat = zeros(1, size(xC, 2));
    for idx = 1:size(xC, 2)
        diff_mat(idx) = min(abs(xC{idx}-gear_rpm) + abs(yC{idx}-gear_torque));
    end
    [~, idx_min] = min(diff_mat);
    motor_efficiency = zC{idx_min};
    motor_efficiency = sign(gear_torque) * motor_efficiency;
